simulink model "flightController"  (R2018b)
settings: Solver=ode3  StartTime=0  StopTime=35  FixedStep=Ts  RelTol=1e-3  EnableMultiTasking=on
undefined symbols (not defined in the file): Controller, DiscIntNeverNeededParam, g, Ts, Vehicle
settings Model: ExtModeTrigDuration=80  Creator=The MathWorks, Inc.  LastModifiedBy=TOSHIBA
settings SolverCC: MinimalZcImpactIntegration=on
settings DataIOCC: LimitDataPoints=on  SaveFormat=Array
settings OptimizationCC: BlockReduction=off  EnhancedBackFolding=on  PassReuseOutputArgsAs=Individual arguments  MaxStackSize=64  OptimizeBlockOrder=speed  DifferentSizesBufferReuse=on  OptimizationCustomize=off
settings DebuggingCC: AlgebraicLoopMsg=none  ParameterPrecisionLossMsg=none  ParameterTunabilityLossMsg=error  UnconnectedInputMsg=none  UnconnectedOutputMsg=none  UnconnectedLineMsg=none  BusObjectLabelMismatch=error  LibraryContextMissingDiagnostic=none  SFUnexpectedBacktrackingDiag=warning  SFNoUnconditionalDefaultTransitionDiag=warning  SFExecutionAtInitializationDiag=none
settings HardwareCC: ProdBitPerPointer=32  ProdBitPerSizeT=32  ProdBitPerPtrDiffT=32  ProdLargestAtomicInteger=Long  ProdWordSize=32  ProdHWDeviceType=ARM Compatible->ARM 9
settings ModelReferenceCC: ModelReferenceNumInstancesAllowed=Single  PropagateSignalLabelsOutOfModel=off
settings SFSimCC: SimUseLocalCustomCode=off  MATLABDynamicMemAlloc=off
settings RTWCC: SystemTargetFile=ert.tlc  HardwareBoard=PARROT Mambo  TemplateMakefile=ert_default_tmf  GenerateReport=on  RTWUseLocalCustomCode=off  Toolchain=Sourcery G++ Lite GNU Toolchain for Drones  IncludeHyperlinkInReport=on  LaunchReport=on  GenerateTraceInfo=on  GenerateTraceReport=on  GenerateTraceReportSl=on  GenerateTraceReportSf=on  GenerateTraceReportEml=on
settings CodeAppCC: ForceParamTrailComments=on  IgnoreCustomStorageClasses=off  MaxIdLength=63  OperatorAnnotations=on  SimulinkDataObjDesc=on  SFDataObjDesc=on  InsertBlockDesc=on
settings ConfigComp: CovMetricSettings=dw  CovHtmlReporting=on  CovSaveCumulativeToWorkspaceVar=on  CovSaveSingleToWorkspaceVar=on  CovExternalEMLEnable=off  CovSFcnEnable=off

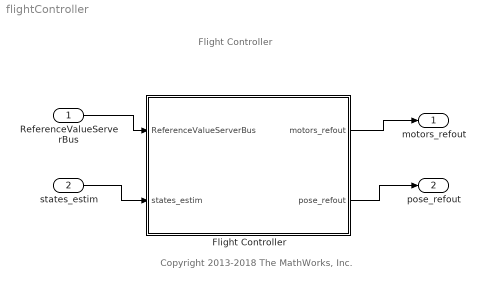
== system flightController ==
  note: Flight Controller
  note: Copyright 2013-2018 The MathWorks, Inc.
  ReferenceValueServerBus : Inport  OutDataTypeStr=Bus: CommandBus  BusOutputAsStruct=on
  states_estim : Inport  Port=2  OutDataTypeStr=Bus: statesEstim_t  BusOutputAsStruct=on
  Flight Controller : Subsystem
  motors_refout : Outport
  pose_refout : Outport  Port=2
  wires:
  ReferenceValueServerBus/1 -> Flight Controller/1(ReferenceValueServerBus)
  states_estim/1 -> Flight Controller/2(states_estim)
  Flight Controller/2(pose_refout) -> pose_refout/1
  Flight Controller/1(motors_refout) -> motors_refout/1

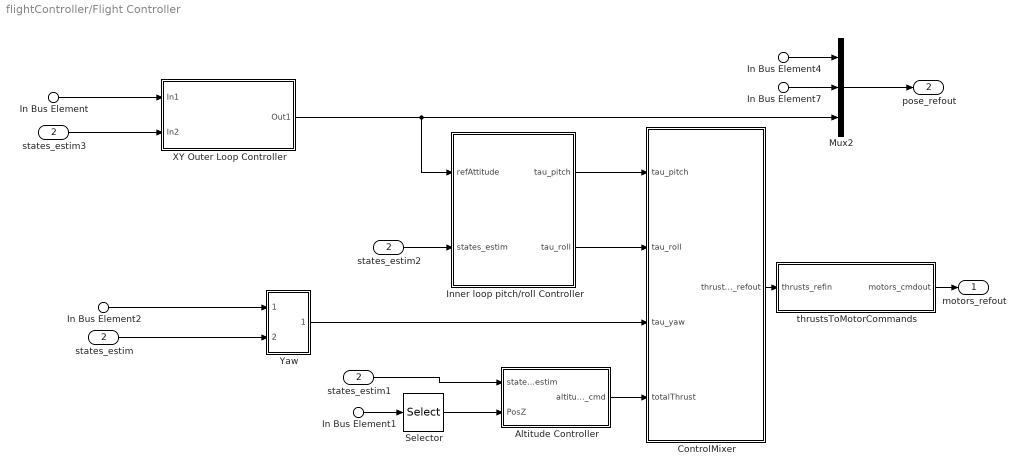
== system flightController/Flight Controller ==
  In Bus Element : Inport  PortName=ReferenceValueServerBus  Element=pos_ref
  In Bus Element4 : Inport  PortName=ReferenceValueServerBus  Element=pos_ref
  In Bus Element1 : Inport  PortName=ReferenceValueServerBus  Element=pos_ref
  In Bus Element2 : Inport  PortName=ReferenceValueServerBus  Element=orient_ref
  In Bus Element7 : Inport  PortName=ReferenceValueServerBus  Element=orient_ref
  states_estim : Inport  Port=2
  Altitude Controller : Subsystem
  ControlMixer : Subsystem
  Inner loop pitch/roll Controller : Subsystem
  Mux2 : Mux  Inputs=3
  Selector : Selector  InputPortWidth=3  IndexOptions=Index vector (dialog)  Indices=3  OutputSizes=1
  "XY Outer Loop Controller " : Subsystem
  Yaw : Subsystem
  states_estim1 : InportShadow  Port=2
  states_estim2 : InportShadow  Port=2
  states_estim3 : InportShadow  Port=2
  thrustsToMotorCommands : Subsystem
  motors_refout : Outport
  pose_refout : Outport  Port=2
  wires:
  thrustsToMotorCommands/1(motors_cmdout) -> motors_refout/1
  ControlMixer/1(thrusts_refout) -> thrustsToMotorCommands/1(thrusts_refin)
  Altitude Controller/1(altitude_cmd) -> ControlMixer/4(totalThrust)
  Mux2/1 -> pose_refout/1
  Inner loop pitch/roll Controller/1(tau_pitch) -> ControlMixer/1(tau_pitch)
  Inner loop pitch/roll Controller/2(tau_roll) -> ControlMixer/2(tau_roll)
  states_estim1/1 -> Altitude Controller/1(states_estim)
  states_estim2/1 -> Inner loop pitch/roll Controller/2(states_estim)
  In Bus Element4/1 -> Mux2/1
  In Bus Element7/1 -> Mux2/2
  "XY Outer Loop Controller "/1(Out1) -> Inner loop pitch/roll Controller/1(refAttitude), Mux2/3
  In Bus Element/1 -> "XY Outer Loop Controller "/1(In1)
  states_estim3/1 -> "XY Outer Loop Controller "/2(In2)
  In Bus Element2/1 -> Yaw/1(In1)
  states_estim/1 -> Yaw/2(In2)
  Yaw/1(Out1) -> ControlMixer/3(tau_yaw)
  In Bus Element1/1 -> Selector/1
  Selector/1 -> Altitude Controller/2(PosZ)

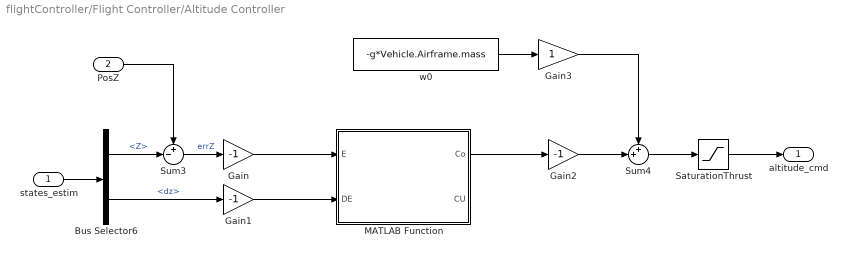
== system flightController/Flight Controller/Altitude Controller ==
  states_estim : Inport
  PosZ : Inport  Port=2
  Bus Selector6 : BusSelector  OutputSignals=Z,dz
  Gain : Gain  Gain=-1
  Gain1 : Gain  Gain=-1
  Gain2 : Gain  Gain=-1
  Gain3 : Gain
  MATLAB Function : MATLAB Function  TreatAsAtomicUnit=on
  SaturationThrust : Saturate  UpperLimit=4*Controller.totalThrustMaxRelative*Controller.motorsThrustPerMotorMax  LowerLimit=-4*Controller.totalThrustMaxRelative*Controller.motorsThrustPerMotorMax  OutDataTypeStr=single
  Sum3 : Sum  Inputs=+-|  AccumDataTypeStr=single  OutDataTypeStr=single  SaturateOnIntegerOverflow=on
  Sum4 : Sum  Inputs=++|  AccumDataTypeStr=single  OutDataTypeStr=single  SaturateOnIntegerOverflow=on
  w0 : Constant  Value=-g*Vehicle.Airframe.mass  OutDataTypeStr=single  SampleTime=Ts
  altitude_cmd : Outport
  wires:
  Sum3/1 -> Gain/1  "errZ"
  Bus Selector6/1 -> Sum3/2  "<Z>"
  Bus Selector6/2 -> Gain1/1  "<dz>"
  w0/1 -> Gain3/1
  PosZ/1 -> Sum3/1
  states_estim/1 -> Bus Selector6/1
  Gain2/1 -> Sum4/2
  Sum4/1 -> SaturationThrust/1
  SaturationThrust/1 -> altitude_cmd/1
  Gain/1 -> MATLAB Function/1(E)
  Gain1/1 -> MATLAB Function/2(DE)
  MATLAB Function/1(Co) -> Gain2/1
  Gain3/1 -> Sum4/1

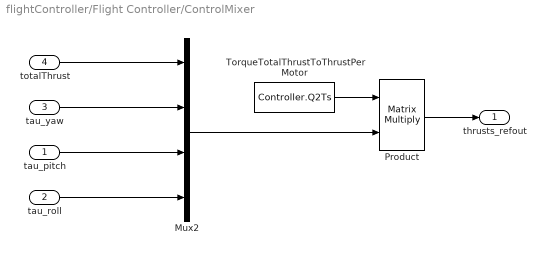
== system flightController/Flight Controller/ControlMixer ==
  tau_pitch : Inport
  tau_roll : Inport  Port=2
  tau_yaw : Inport  Port=3
  totalThrust : Inport  Port=4
  Mux2 : Mux
  Product : Product  Multiplication=Matrix(*)  RndMeth=Zero
  TorqueTotalThrustToThrustPerMotor : Constant  Value=Controller.Q2Ts  OutDataTypeStr=single
  thrusts_refout : Outport
  wires:
  Product/1 -> thrusts_refout/1
  tau_roll/1 -> Mux2/4
  tau_pitch/1 -> Mux2/3
  tau_yaw/1 -> Mux2/2
  totalThrust/1 -> Mux2/1
  TorqueTotalThrustToThrustPerMotor/1 -> Product/1
  Mux2/1 -> Product/2

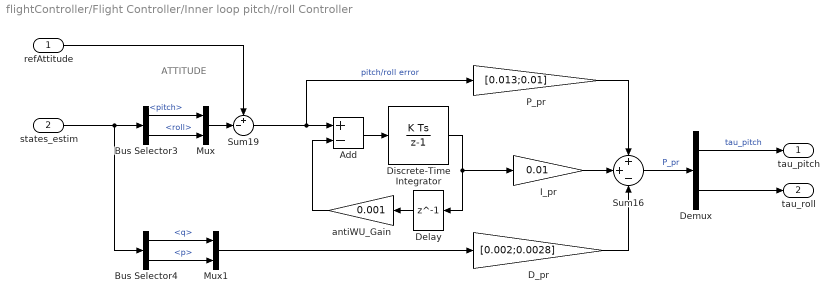
== system flightController/Flight Controller/Inner loop pitch//roll Controller ==
  note: ATTITUDE
  refAttitude : Inport
  states_estim : Inport  Port=2
  Add : Sum  Inputs=+-
  Bus Selector3 : BusSelector  OutputSignals=pitch,roll
  Bus Selector4 : BusSelector  OutputSignals=q,p
  D_pr : Gain  Gain=[0.002;0.0028]
  Delay : Delay  DelayLength=1  InitialCondition=0
  Demux : Demux  Outputs=2
  Discrete-Time Integrator : DiscreteIntegrator  SampleTime=Ts  LimitOutput=on  UpperSaturationLimit=2  LowerSaturationLimit=-2  ICPrevOutput=DiscIntNeverNeededParam  ICPrevScaledInput=DiscIntNeverNeededParam
  I_pr : Gain  Gain=0.01
  Mux : Mux  Inputs=2
  Mux1 : Mux  Inputs=2
  P_pr : Gain  Gain=[0.013;0.01]
  Sum16 : Sum  Inputs=++-  AccumDataTypeStr=single  OutDataTypeStr=single  SaturateOnIntegerOverflow=on
  Sum19 : Sum  Inputs=+-|
  antiWU_Gain : Gain  Gain=0.001
  tau_pitch : Outport
  tau_roll : Outport  Port=2
  wires:
  Sum16/1 -> Demux/1  "P_pr"
  antiWU_Gain/1 -> Add/2
  Add/1 -> Discrete-Time Integrator/1
  Bus Selector3/1 -> Mux/1  "<pitch>"
  Bus Selector4/1 -> Mux1/1  "<q>"
  P_pr/1 -> Sum16/1
  I_pr/1 -> Sum16/2
  Sum19/1 -> Add/1, P_pr/1  "pitch/roll error"
  Discrete-Time Integrator/1 -> Delay/1, I_pr/1
  Delay/1 -> antiWU_Gain/1
  Demux/1 -> tau_pitch/1  "tau_pitch"
  Demux/2 -> tau_roll/1
  D_pr/1 -> Sum16/3
  states_estim/1 -> Bus Selector3/1, Bus Selector4/1
  refAttitude/1 -> Sum19/1
  Mux/1 -> Sum19/2
  Bus Selector3/2 -> Mux/2  "<roll>"
  Mux1/1 -> D_pr/1
  Bus Selector4/2 -> Mux1/2  "<p>"

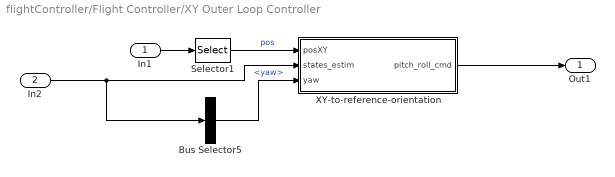
== system flightController/Flight Controller/XY Outer Loop Controller  ==
  In1 : Inport
  In2 : Inport  Port=2
  Bus Selector5 : BusSelector  OutputSignals=yaw
  Selector1 : Selector  InputPortWidth=3  IndexOptions=Index vector (dialog)  Indices=[1 2]  OutputSizes=1
  XY-to-reference-orientation : Subsystem
  Out1 : Outport
  wires:
  In2/1 -> Bus Selector5/1, XY-to-reference-orientation/2(states_estim)
  Selector1/1 -> XY-to-reference-orientation/1(posXY)  "pos"
  Bus Selector5/1 -> XY-to-reference-orientation/3(yaw)  "<yaw>"
  In1/1 -> Selector1/1
  XY-to-reference-orientation/1(pitch_roll_cmd) -> Out1/1

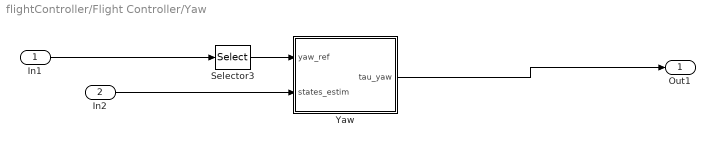
== system flightController/Flight Controller/Yaw ==
  In1 : Inport
  In2 : Inport  Port=2
  Selector3 : Selector  InputPortWidth=3  IndexOptions=Index vector (dialog)  Indices=1  OutputSizes=1
  Yaw : Subsystem
  Out1 : Outport
  wires:
  Selector3/1 -> Yaw/1(yaw_ref)
  In2/1 -> Yaw/2(states_estim)
  In1/1 -> Selector3/1
  Yaw/1(tau_yaw) -> Out1/1

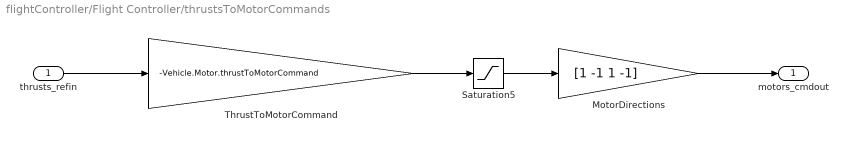
== system flightController/Flight Controller/thrustsToMotorCommands ==
  thrusts_refin : Inport
  MotorDirections : Gain  Gain=[1 -1 1 -1]
  Saturation5 : Saturate  UpperLimit=Vehicle.Motor.maxLimit  LowerLimit=Vehicle.Motor.minLimit
  ThrustToMotorCommand : Gain  Gain=-Vehicle.Motor.thrustToMotorCommand
  motors_cmdout : Outport
  wires:
  Saturation5/1 -> MotorDirections/1
  MotorDirections/1 -> motors_cmdout/1
  ThrustToMotorCommand/1 -> Saturation5/1
  thrusts_refin/1 -> ThrustToMotorCommand/1

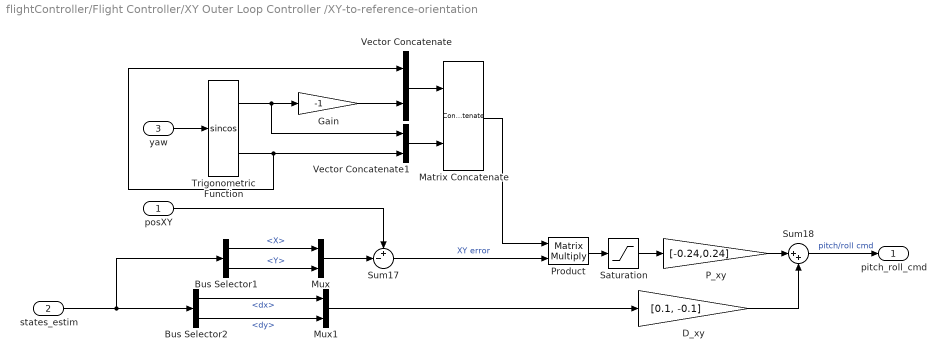
== system flightController/Flight Controller/XY Outer Loop Controller /XY-to-reference-orientation ==
  posXY : Inport
  states_estim : Inport  Port=2
  yaw : Inport  Port=3
  Bus Selector1 : BusSelector  OutputSignals=X,Y
  Bus Selector2 : BusSelector  OutputSignals=dx,dy
  D_xy : Gain  Gain=[0.1, -0.1]  ParamDataTypeStr=single  OutDataTypeStr=single  SaturateOnIntegerOverflow=on
  Gain : Gain  Gain=-1
  Matrix Concatenate : Concatenate  Mode=Multidimensional array  ConcatenateDimension=2
  Mux : Mux  Inputs=2
  Mux1 : Mux  Inputs=2
  P_xy : Gain  Gain=[-0.24,0.24]  ParamDataTypeStr=single  OutDataTypeStr=single  SaturateOnIntegerOverflow=on
  Product : Product  Multiplication=Matrix(*)  OutDataTypeStr=single  RndMeth=Zero
  Saturation : Saturate  UpperLimit=3  LowerLimit=-3  OutDataTypeStr=single
  Sum17 : Sum  Inputs=+-|  AccumDataTypeStr=single
  Sum18 : Sum  Inputs=|++  AccumDataTypeStr=single  OutDataTypeStr=single  SaturateOnIntegerOverflow=on
  Trigonometric Function : Trigonometry  Operator=sincos
  Vector Concatenate : Concatenate
  Vector Concatenate1 : Concatenate
  pitch_roll_cmd : Outport
  wires:
  yaw/1 -> Trigonometric Function/1
  Saturation/1 -> P_xy/1
  P_xy/1 -> Sum18/1
  Sum17/1 -> Product/2  "XY error"
  posXY/1 -> Sum17/1
  Bus Selector2/1 -> Mux1/1  "<dx>"
  states_estim/1 -> Bus Selector2/1, Bus Selector1/1
  Sum18/1 -> pitch_roll_cmd/1  "pitch/roll cmd"
  D_xy/1 -> Sum18/2
  Bus Selector1/1 -> Mux/1  "<X>"
  Product/1 -> Saturation/1
  Trigonometric Function/1 -> Gain/1, Vector Concatenate1/1
  Trigonometric Function/2 -> Vector Concatenate1/2, Vector Concatenate/1
  Gain/1 -> Vector Concatenate/2
  Vector Concatenate/1 -> Matrix Concatenate/1
  Vector Concatenate1/1 -> Matrix Concatenate/2
  Matrix Concatenate/1 -> Product/1
  Bus Selector1/2 -> Mux/2  "<Y>"
  Mux/1 -> Sum17/2
  Mux1/1 -> D_xy/1
  Bus Selector2/2 -> Mux1/2  "<dy>"

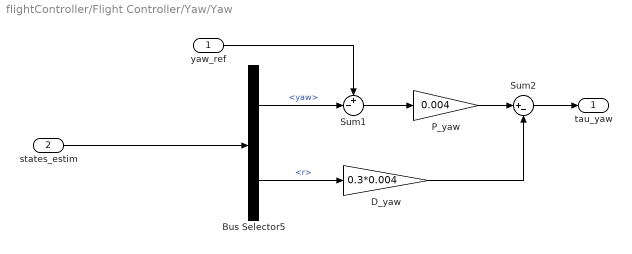
== system flightController/Flight Controller/Yaw/Yaw ==
  yaw_ref : Inport
  states_estim : Inport  Port=2
  Bus Selector5 : BusSelector  OutputSignals=yaw,r
  D_yaw : Gain  Gain=0.3*0.004
  P_yaw : Gain  Gain=0.004  ParamDataTypeStr=single  OutDataTypeStr=single
  Sum1 : Sum  Inputs=+-|  AccumDataTypeStr=single  OutDataTypeStr=single  SaturateOnIntegerOverflow=on
  Sum2 : Sum  Inputs=|+-
  tau_yaw : Outport
  wires:
  D_yaw/1 -> Sum2/2
  P_yaw/1 -> Sum2/1
  Bus Selector5/2 -> D_yaw/1  "<r>"
  Sum1/1 -> P_yaw/1
  states_estim/1 -> Bus Selector5/1
  Sum2/1 -> tau_yaw/1
  Bus Selector5/1 -> Sum1/2  "<yaw>"
  yaw_ref/1 -> Sum1/1

== matlab function flightController/Flight Controller/Altitude Controller/MATLAB Function ==
  data: E input; Co output; DE input; CU output
function [Co, CU] = controller_fuzzy3(E, DE)

C = [[0,0,-0.2;1,1,0.2;0,1,-.45;1,0,0.45;0.50,0.50,0.0;0,0.38127,-0.66;0.311,0,0.220;0.9732,0.5819,0.660;0.6421,0.9832,-0.280;0.4816,0,0.50;0.4515,0.993,-0.590;0,0.5418,-0.830;0.9732,0.3812,0.880;0.5618,0,0.620;0.2709,0.5819,-0.450;0,0.6321,-0.930;0.6020,0.2842,0.390;0.6120,0,0.70;0.6822,0,0.820;0.3311,0.9732,-0.760;0,0.1137,-0.380;0.9732,0.2842,0.980;0.9732,0,1.280;0.9832,0.8026,0.450;0,0.6822,-0.980;0,0.9832,-1.3]];

%Normalizing the inputs to 0-1 interval
EN = (E - (-1.1))/2 ;
DEN = (DE - (-1.77))/3;

%mu=0.3;
%mu1= (1-mu)/mu;

mu=[0.358,0.3549,0.3568,0.3568,0.3549,0.1274,0.1883,0.1743,0.2311,0.050,0.05,0.05,0.05,0.05,0.05,0.05,.05,0.05,0.05,0.05,0.05,0.05,0.05,0.05,0.05,0.05];
mu1= (1-mu)./mu;


lambda = 4;
e = 0.33;
Noise=0.1;       %0.05;

G11U = zeros(size(C(:,1)));
G11L = zeros(size(C(:,1)));
G12U = zeros(size(C(:,1)));
G12L = zeros(size(C(:,1)));
RU = zeros(size(C(:,1)));
RL = zeros(size(C(:,1)));

for i= 1: length(C(:,1))
    
% 1st input type2 Membership function
deltal1 = abs(((EN-(C(i,1)))/ e ) * (1 / (1 + exp(100*((EN-(C(i,1))))))))^lambda;
deltar1 = abs(((EN-(C(i,1)))/ e ) * (1 / (1 + exp(-100*((EN-(C(i,1))))))))^lambda;
G11U(i) = 1/(1+ (mu1(i) * deltal1) + (mu1(i) *deltar1));

deltal2 = abs((((EN-(C(i,1)))- Noise)/ (e) ) * (1 / (1 + exp(100*(((EN-(C(i,1)))- Noise))))))^(lambda);
deltar2 = abs((((EN-(C(i,1)))+ Noise)/ (e) ) * (1 / (1 + exp(-100*(((EN-(C(i,1)))+ Noise))))))^(lambda);
G11L(i) = 1/(1+ (mu1(i) * deltal2) + (mu1(i) *deltar2));

% 2nd Input type2 Membership function
deltal1 = abs(((DEN-(C(i,2)))/ e ) * (1 / (1 + exp(100*((DEN-(C(i,2))))))))^lambda;
deltar1 = abs(((DEN-(C(i,2)))/ e ) * (1 / (1 + exp(-100*((DEN-(C(i,2))))))))^lambda;
G12U(i) = 1/(1+ (mu1(i) * deltal1) + (mu1(i) *deltar1));
 
deltal2 = abs((((DEN-(C(i,2)))- Noise)/ (e) ) * (1 / (1 + exp(100*(((DEN-(C(i,2)))- Noise))))))^(lambda);
deltar2 = abs((((DEN-(C(i,2)))+ Noise)/ (e) ) * (1 / (1 + exp(-100*(((DEN-(C(i,2)))+ Noise))))))^(lambda);
G12L(i) = 1/(1+ (mu1(i) * deltal2) + (mu1(i) *deltar2));

end

for i= 1: length(C(:,1))
    
RU(i) = 1/(((1-G11U(i))/G11U(i)) + ((1-G12U(i))/G12U(i)));
RL(i) = 1/(((1-G11L(i))/G11L(i)) + ((1-G12L(i))/G12L(i)));   
   
end

RUN = RU/(sum(RU));
RLN = RL/(sum(RL));

CU = dot(RUN,C(:,3));
CL = dot(RLN,C(:,3));
Co = ((CU + CL) / 2) ;

end
